simulink model "visual_line_follower_sac_lyapunov_gazebo"  (R2026a)
settings: Solver=FixedStepDiscrete  StopTime=inf  FixedStep=Ts_Control  EnableMultiTasking=on
InitFcn:
  | run(fullfile(fileparts(get_param(bdroot,"FileName")),"runtime","configure_visual_line_follower_gazebo_debug.m"));
model workspace (MAT data in the model file):
  BaseLinearSpeed = 20
  BaseSpeedScale = 0.03
  Kd_Line = 0.35
  Ki_Line = 0
  Kp_Line = 5
  LocalPath_CurvatureGain = 0.04
  LocalPath_HeadingGain = 0.35
  LocalPath_LateralGain = 0.6
  LocalPath_LookaheadDistance = 0.72
  LocalPath_NumPoints = 30
  LocalPath_ROIFraction = 0.1
  MJ_StepTime = 0.002
  MJ_TargetLateralPosition = 0
  MaxAngularSpeed = 1.5
  MaxWheelSpeed = 25
  N_Line = 20
  OriginBot_ErrorScale = 500
  OriginBot_MaxSaturation = 0.3
  OriginBot_MinBrightness = 70
  OriginBot_MinPixels = 30
  OriginBot_ROIHeight = 45
  OriginBot_ROIStartFraction = 0.72
  SAC_Done_Steps = 100
  SAC_Eps = 0.001
  SAC_K_inv = 0.1
  SAC_Lambda = 0.5
  SAC_MaxDeltaOmega = 1
  SAC_P_Lost = 10
  SAC_Q = 1
  SAC_Q_e = 1
  SAC_Q_h = 1
  SAC_Q_l = 1
  SAC_R = 0.1
  SL_ROS_VariableLengthArrays_MaxSizes.CommonInfo.ArrayTruncateAction = 'EmitWarning'
  SL_ROS_VariableLengthArrays_MaxSizes.MsgTypeMap = containers.Map
  SL_ROS_VariableLengthArrays_MaxSizes.MsgTypeMap.serialization.keys = {'sensor_msgs/Image'}
  SL_ROS_VariableLengthArrays_MaxSizes.MsgTypeMap.serialization.values{1}(1).PropertyName = 'data'
  SL_ROS_VariableLengthArrays_MaxSizes.MsgTypeMap.serialization.values{1}(1).DataType = 'uint8'
  SL_ROS_VariableLengthArrays_MaxSizes.MsgTypeMap.serialization.values{1}(1).MaxLength = 6220800
  SL_ROS_VariableLengthArrays_MaxSizes.MsgTypeMap.serialization.values{1}(2).PropertyName = 'encoding'
  SL_ROS_VariableLengthArrays_MaxSizes.MsgTypeMap.serialization.values{1}(2).DataType = 'uint8'
  SL_ROS_VariableLengthArrays_MaxSizes.MsgTypeMap.serialization.values{1}(2).MaxLength = 128
  SL_ROS_VariableLengthArrays_MaxSizes.MsgTypeMap.serialization.uniformity = 0
  SL_ROS_VariableLengthArrays_MaxSizes.MsgTypeMap.serialization.keyType = 'char'
  SL_ROS_VariableLengthArrays_MaxSizes.MsgTypeMap.serialization.valueType = 'any'
  SteeringSign = 1
  TB3_WheelRadius = 0.033
  TB3_WheelSeparation = 0.288
  Ts_Control = 0.05
  Ts_Stop = 10
  Ts_Vision = 0.05
  TurtleBot3MuJoCoMap = "complex"
  TurtleBot3MuJoCoScene = ""
  k_heading = 0.55
undefined symbols (not defined in the file): angular, linear, originbot_line_follower_debug_frame_gazebo, originbot_local_path_generator_gazebo
libraries: ros2lib x4, slpidlib x1, rllib x1
settings Model: ExtModeTrigDuration=10000  Creator=HP  LastModifiedBy=kevin
settings SolverCC: PositivePriorityOrder=on
settings ConfigComp: CovMetricSettings=dswe

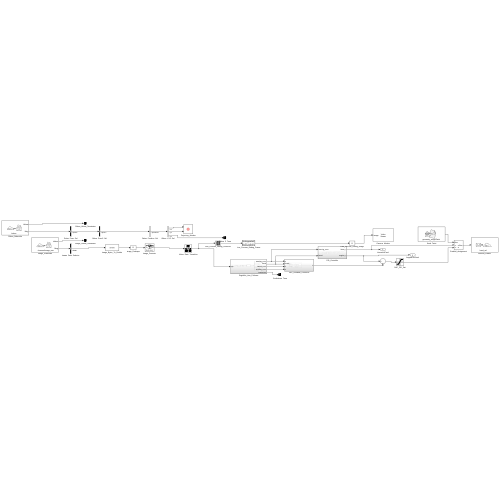
[thumbnail: Simulink's stored preview of the top-level diagram]
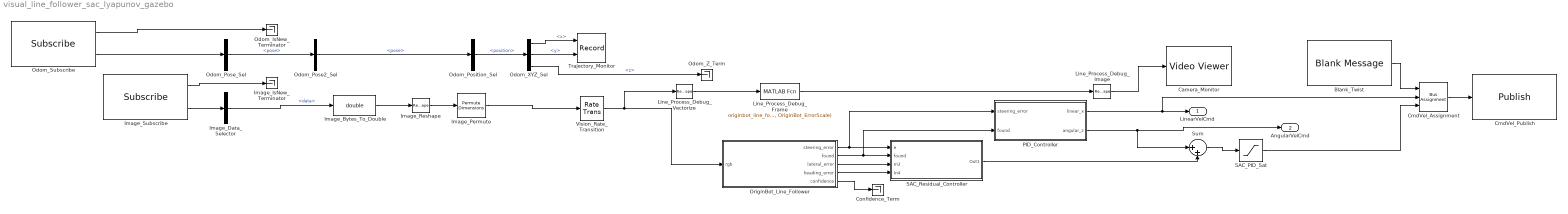
== system visual_line_follower_sac_lyapunov_gazebo ==
  Blank_Twist : ros2lib/Blank Message  messageClass=Message  entityType=geometry_msgs/Twist  messageType=geometry_msgs/Twist  SampleTime=inf
  Camera_Monitor : VideoViewer  FigPos=[2041 741 418 304]
  CmdVel_Assignment : BusAssignment  AssignedSignals=linear.x,angular.z
  CmdVel_Publish : ros2lib/Publish  topicSource=Select from ROS network  topic=/cmd_vel  messageType=geometry_msgs/Twist  QOSHistory=Keep last  QOSDepth=10  QOSReliability=Reliable  QOSDurability=Volatile  QOSDeadline=Inf  QOSLifespan=Inf  QOSLiveliness=Automatic  QOSLeaseDuration=Inf  QOSAvoidROSNamespaceConventions=off
  Confidence_Term : Terminator
  Image_Bytes_To_Double : DataTypeConversion  OutDataTypeStr=double
  Image_Data_Selector : BusSelector  OutputSignals=data
  Image_IsNew_Terminator : Terminator
  Image_Permute : PermuteDimensions  Order=[3 2 1]
  Image_Reshape : Reshape  OutputDimensionality=Customize  OutputDimensions=[3,1920,1080]
  Image_Subscribe : ros2lib/Subscribe  topicSource=Select from ROS network  topic=/camera/image_raw  messageType=sensor_msgs/Image  sampleTime=Ts_Vision  QOSHistory=Keep last  QOSDepth=10  QOSReliability=Reliable  QOSDurability=Volatile  QOSDeadline=Inf  QOSLifespan=Inf  QOSLiveliness=Automatic  QOSLeaseDuration=Inf  QOSAvoidROSNamespaceConventions=off
  Line_Process_Debug_Frame : MATLABFcn  MATLABFcn=originbot_line_follower_debug_frame_gazebo(u, LocalPath_ROIFraction, LocalPath_NumPoints, OriginBot_MinBrightness, OriginBot_MaxSaturation, OriginBot_MinPixels, OriginBot_ErrorScale)
  Line_Process_Debug_Image : Reshape  OutputDimensionality=Customize  OutputDimensions=[1080,1920,3]
  Line_Process_Debug_Vectorize : Reshape  OutputDimensionality=Column vector (2-D)
  Odom_IsNew_Terminator : Terminator
  Odom_Pose2_Sel : BusSelector  OutputSignals=pose
  Odom_Pose_Sel : BusSelector  OutputSignals=pose
  Odom_Position_Sel : BusSelector  OutputSignals=position
  Odom_Subscribe : ros2lib/Subscribe  topicSource=Select from ROS network  topic=/odom  messageType=nav_msgs/Odometry  sampleTime=Ts_Control  QOSHistory=Keep last  QOSDepth=10  QOSReliability=Reliable  QOSDurability=Volatile  QOSDeadline=Inf  QOSLifespan=Inf  QOSLiveliness=Automatic  QOSLeaseDuration=Inf  QOSAvoidROSNamespaceConventions=off
  Odom_XYZ_Sel : BusSelector  OutputSignals=x,y,z
  Odom_Z_Term : Terminator
  OriginBot_Line_Follower : Subsystem
  PID_Controller : Subsystem
  SAC_PID_Sat : Saturate  UpperLimit=2*MaxWheelSpeed*TB3_WheelRadius/TB3_WheelSeparation  LowerLimit=-2*MaxWheelSpeed*TB3_WheelRadius/TB3_WheelSeparation
  SAC_Residual_Controller : Subsystem
  Sum : Sum  Inputs=|++
  Trajectory_Monitor : Record  NumPorts=2.0  FileSettingsInternal="{\"entries\":[{\"content\":{\"excelSettings\":{\"content\":{},\"type\":\"Streamout.ExcelSettings\"},\"parquetSettings\":{\"content\":{},\"type\":\"Streamout.ParquetSettings\"}},\"type\":\"Streamout.FileSettingStorage\",\"uuid\":\"\"}],\"packageUris\":[\"http:\\/\\/schema.mathworks.com\\/mf0\\/streamout_blocks\\/R2020a\"],\"version\":\"1.0\"}"  FrameSettings=[0, 0]  SignalsInternal="{\"entries\":[{\"content\":{},\"type\":\"RecordBlkView.InputSignals\",\"uuid\":\"\"}],\"packageUris\":[\"http:\\/\\/schema.mathworks.com\\/mf0\\/streamout_blocks\\/R2020a\"],\"version\":\"1.0\"}"  VisualizationBindings="{\"sparklinesplugin\":{\"info\":[{\"bindingParametersList\":[],\"subplotID\":1}]}}"
  Vision_Rate_Transition : RateTransition
  LinearVelCmd : Outport
  AngularVelCmd : Outport  Port=2
  wires:
  SAC_PID_Sat/1 -> CmdVel_Assignment/3
  Line_Process_Debug_Image/1 -> Camera_Monitor/1
  Line_Process_Debug_Frame/1 -> Line_Process_Debug_Image/1
  Line_Process_Debug_Vectorize/1 -> Line_Process_Debug_Frame/1
  Image_Permute/1 -> Vision_Rate_Transition/1
  Image_Reshape/1 -> Image_Permute/1
  Image_Bytes_To_Double/1 -> Image_Reshape/1
  Image_Data_Selector/1 -> Image_Bytes_To_Double/1  "<data>"
  Image_Subscribe/2 -> Image_Data_Selector/1
  Image_Subscribe/1 -> Image_IsNew_Terminator/1
  Sum/1 -> SAC_PID_Sat/1
  SAC_Residual_Controller/1(Out1) -> Sum/2
  PID_Controller/2(angular_z) -> Sum/1, AngularVelCmd/1
  PID_Controller/1(linear_x) -> LinearVelCmd/1, CmdVel_Assignment/2
  Blank_Twist/1 -> CmdVel_Assignment/1
  CmdVel_Assignment/1 -> CmdVel_Publish/1
  Odom_Subscribe/1 -> Odom_IsNew_Terminator/1
  Odom_Subscribe/2 -> Odom_Pose_Sel/1
  Odom_Pose_Sel/1 -> Odom_Pose2_Sel/1  "<pose>"
  Odom_Pose2_Sel/1 -> Odom_Position_Sel/1  "<pose>"
  Odom_Position_Sel/1 -> Odom_XYZ_Sel/1  "<position>"
  Odom_XYZ_Sel/3 -> Odom_Z_Term/1  "<z>"
  Odom_XYZ_Sel/1 -> Trajectory_Monitor/1  "<x>"
  Odom_XYZ_Sel/2 -> Trajectory_Monitor/2  "<y>"
  Vision_Rate_Transition/1 -> OriginBot_Line_Follower/1(rgb), Line_Process_Debug_Vectorize/1
  OriginBot_Line_Follower/1(steering_error) -> SAC_Residual_Controller/1(e), PID_Controller/1(steering_error)
  OriginBot_Line_Follower/2(found) -> SAC_Residual_Controller/2(found), PID_Controller/2(found)
  OriginBot_Line_Follower/3(lateral_error) -> SAC_Residual_Controller/3(In3)
  OriginBot_Line_Follower/4(heading_error) -> SAC_Residual_Controller/4(In4)
  OriginBot_Line_Follower/5(confidence) -> Confidence_Term/1

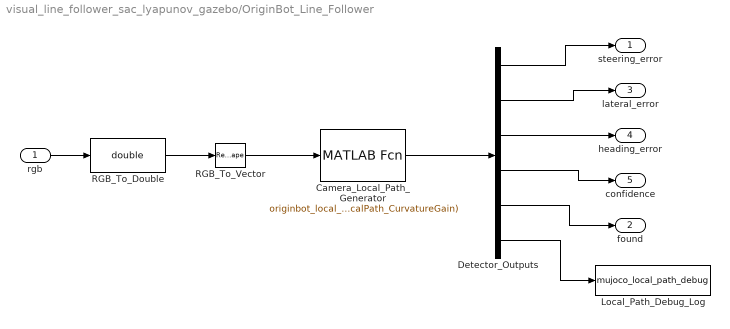
== system visual_line_follower_sac_lyapunov_gazebo/OriginBot_Line_Follower ==
  rgb : Inport
  Camera_Local_Path_Generator : MATLABFcn  MATLABFcn=originbot_local_path_generator_gazebo(u, LocalPath_ROIFraction, LocalPath_NumPoints, OriginBot_MinBrightness, OriginBot_MaxSaturation, OriginBot_MinPixels, OriginBot_ErrorScale, LocalPath_LookaheadDistance, LocalPath_LateralGain, LocalPath_HeadingGain, LocalPath_CurvatureGain)  OutputDimensions=72  OutputSignalType=real  SampleTime=Ts_Vision
  Detector_Outputs : Demux  Outputs=[1 1 1 1 1 67]
  Local_Path_Debug_Log : ToWorkspace  VariableName=mujoco_local_path_debug  SaveFormat=Timeseries  SampleTime=-1
  RGB_To_Double : DataTypeConversion  OutDataTypeStr=double
  RGB_To_Vector : Reshape  OutputDimensionality=Column vector (2-D)
  steering_error : Outport
  found : Outport  Port=2
  lateral_error : Outport  Port=3
  heading_error : Outport  Port=4
  confidence : Outport  Port=5
  wires:
  Detector_Outputs/6 -> Local_Path_Debug_Log/1
  Detector_Outputs/5 -> found/1
  Detector_Outputs/3 -> heading_error/1
  Detector_Outputs/1 -> steering_error/1
  Camera_Local_Path_Generator/1 -> Detector_Outputs/1
  Detector_Outputs/4 -> confidence/1
  RGB_To_Vector/1 -> Camera_Local_Path_Generator/1
  RGB_To_Double/1 -> RGB_To_Vector/1
  rgb/1 -> RGB_To_Double/1
  Detector_Outputs/2 -> lateral_error/1

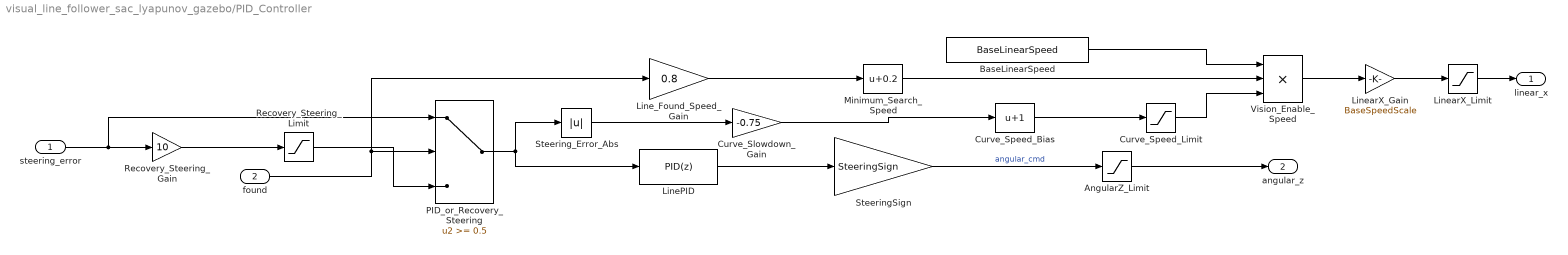
== system visual_line_follower_sac_lyapunov_gazebo/PID_Controller ==
  steering_error : Inport
  found : Inport  Port=2
  AngularZ_Limit : Saturate  UpperLimit=2*MaxWheelSpeed*TB3_WheelRadius/TB3_WheelSeparation  LowerLimit=-2*MaxWheelSpeed*TB3_WheelRadius/TB3_WheelSeparation
  BaseLinearSpeed : Constant  Value=BaseLinearSpeed
  Curve_Slowdown_Gain : Gain  Gain=-0.75
  Curve_Speed_Bias : Bias  Bias=1
  Curve_Speed_Limit : Saturate  UpperLimit=1  LowerLimit=0.25
  LinePID : slpidlib/PID Controller  Controller=PID  Form=Parallel  TimeDomain=Discrete-time  UseExternalTs=off  SampleTime=Ts_Control  IntegratorMethod=Backward Euler  FilterMethod=Trapezoidal  ControllerParametersSource=internal  P=Kp_Line  I=Ki_Line  UseKiTs=off  D=Kd_Line  UseExternalDerivativeSource=off  N=N_Line  UseFilter=on  TunerSelectOption=Transfer Function Based (PID Tuner App)  InitialConditionSource=internal  InitialConditionForIntegrator=0  InitialConditionForFilter=0  DifferentiatorICPrevScaledInput=0  ExternalReset=none  TrackingMode=off  Kt=1  LimitOutput=on  SatLimitsSource=internal  UpperSaturationLimit=MaxAngularSpeed  LowerSaturationLimit=-MaxAngularSpeed  LinearizeAsGain=off  AntiWindupMode=back-calculation  Kb=1  LimitIntegrator=off  UpperIntegratorSaturationLimit=inf  LowerIntegratorSaturationLimit=-inf  POutMin=[]  POutMax=[]  IOutMin=[]  IOutMax=[]  DOutMin=[]  DOutMax=[]  NOutMin=[]  NOutMax=[]  SumOutMin=[]  SumOutMax=[]  SaturationOutMin=[]  SaturationOutMax=[]  PParamMin=[]  PParamMax=[]  IParamMin=[]  IParamMax=[]  DParamMin=[]  DParamMax=[]  NParamMin=[]  NParamMax=[]  KbParamMin=[]  KbParamMax=[]  KtParamMin=[]  KtParamMax=[]  KbOutMin=[]  KbOutMax=[]  KtOutMin=[]  KtOutMax=[]  IntegratorOutMin=[]  IntegratorOutMax=[]  FilterOutMin=[]  FilterOutMax=[]  SumI1OutMin=[]  SumI1OutMax=[]  SumI2OutMin=[]  SumI2OutMax=[]  SumI3OutMin=[]  SumI3OutMax=[]  SumI4OutMin=[]  SumI4OutMax=[]  SumDOutMin=[]  SumDOutMax=[]  DifferentiatorOutMin=[]  DifferentiatorOutMax=[]  FilterDiffOutCoefMin=[]  FilterDiffOutCoefMax=[]  ReciprocalOutMin=[]  ReciprocalOutMax=[]  SumDenOutMin=[]  SumDenOutMax=[]  SumNumOutMin=[]  SumNumOutMax=[]  DivideOutMin=[]  DivideOutMax=[]  UdiffTsProdOutMin=[]  UdiffTsProdOutMax=[]  NTsProdOutMin=[]  NTsProdOutMax=[]  UintegralTsProdOutMin=[]  UintegralTsProdOutMax=[]  UngainTsProdOutMin=[]  UngainTsProdOutMax=[]  ClampingZeroOutDataTypeStr=Inherit: Inherit via back propagation  ClampingZeroOutMin=[]  ClampingZeroOutMax=[]  FilterDenConstantOutDataTypeStr=Inherit: Inherit via back propagation  FilterDenConstantOutMin=[]  FilterDenConstantOutMax=[]  PCopyOutDataTypeStr=Inherit: Inherit via back propagation  PCopyOutMin=[]  PCopyOutMax=[]  NCopyOutDataTypeStr=Inherit: Inherit via back propagation  NCopyOutMin=[]  NCopyOutMax=[]  IntegratorContinuousStateAttributes=''  IntegratorStateMustResolveToSignalObject=off  IntegratorRTWStateStorageClass=Auto  FilterContinuousStateAttributes=''  FilterStateMustResolveToSignalObject=off  FilterRTWStateStorageClass=Auto  ParallelPVariant=InternalParameters  IdealPVariant=Disabled  IVariant=InternalParameters  DVariant=InternalParameters  IntegratorVariant=Discrete  SatVariant=Enabled  AWVariant=BackCalculation  PCopyVariant=Disabled  TRVariant=Disabled  FdbkBlocksVariant=Feedback  IdealPFdbkVariant=Passthrough  SatFdbkVariant=Enabled  DerivativeFilterVariant=TrapezoidalFilter  NVariant=InternalParameters  NCopyVariant=InternalParameters  FilterICVariant=InternalICsFilter  IntegratorICVariant=InternalICs  ExternalResetVariant=Disabled  TRSumVariant=Passthrough  SumFdbkVariant=Enabled  SumVariant=Sum_PID  TsampFilterVariant=InternalTs  TsampNgainVariant=Passthrough  TsampIntegralVariant=Disabled_SignalSpec  ExternalSaturationOutDataTypeStr=Inherit: Same as second input  DerivativeSourceVariant=ErrorSignal  PreIntVariant=InternalPreInt
      settings: LibrarySourceBlock=hdlsllib/Discrete/Discrete PID Controller
  Line_Found_Speed_Gain : Gain  Gain=0.8
  LinearX_Gain : Gain  Gain=BaseSpeedScale
  LinearX_Limit : Saturate  UpperLimit=MaxWheelSpeed*TB3_WheelRadius  LowerLimit=-MaxWheelSpeed*TB3_WheelRadius
  Minimum_Search_Speed : Bias  Bias=0.2
  PID_or_Recovery_Steering : Switch  Threshold=0.5
  Recovery_Steering_Gain : Gain  Gain=10
  Recovery_Steering_Limit : Saturate  UpperLimit=0.45  LowerLimit=-0.45
  SteeringSign : Gain  Gain=SteeringSign
  Steering_Error_Abs : Abs
  Vision_Enable_Speed : Product  Inputs=***
  linear_x : Outport
  angular_z : Outport  Port=2
  wires:
  AngularZ_Limit/1 -> angular_z/1
  SteeringSign/1 -> AngularZ_Limit/1  "angular_cmd"
  LinearX_Limit/1 -> linear_x/1
  LinearX_Gain/1 -> LinearX_Limit/1
  Vision_Enable_Speed/1 -> LinearX_Gain/1
  Curve_Speed_Limit/1 -> Vision_Enable_Speed/3
  BaseLinearSpeed/1 -> Vision_Enable_Speed/1
  LinePID/1 -> SteeringSign/1
  Curve_Speed_Bias/1 -> Curve_Speed_Limit/1
  Curve_Slowdown_Gain/1 -> Curve_Speed_Bias/1
  Steering_Error_Abs/1 -> Curve_Slowdown_Gain/1
  Line_Found_Speed_Gain/1 -> Minimum_Search_Speed/1
  Recovery_Steering_Limit/1 -> PID_or_Recovery_Steering/3
  Recovery_Steering_Gain/1 -> Recovery_Steering_Limit/1
  PID_or_Recovery_Steering/1 -> LinePID/1, Steering_Error_Abs/1
  found/1 -> PID_or_Recovery_Steering/2, Line_Found_Speed_Gain/1
  Minimum_Search_Speed/1 -> Vision_Enable_Speed/2
  steering_error/1 -> PID_or_Recovery_Steering/1, Recovery_Steering_Gain/1

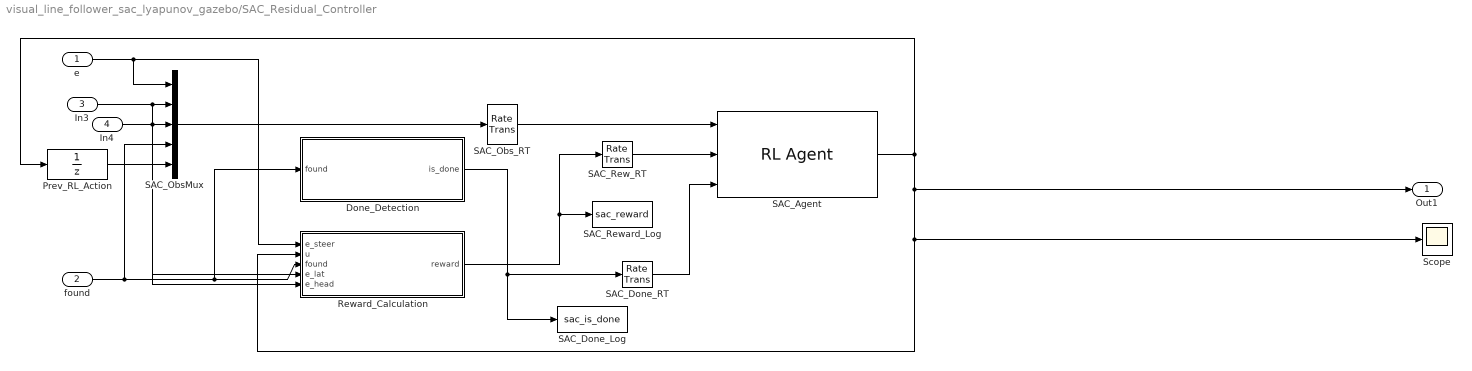
== system visual_line_follower_sac_lyapunov_gazebo/SAC_Residual_Controller ==
  e : Inport
  found : Inport  Port=2
  In3 : Inport  Port=3
  In4 : Inport  Port=4
  Done_Detection : Subsystem
  Prev_RL_Action : UnitDelay  SampleTime=Ts_Control
  Reward_Calculation : Subsystem
  SAC_Agent : rllib/RL Agent  Agent=trainedAgent  ExternalActionAsInput=off  ProvideLastAction=off  ProvideCumRwd=off  TreatAsDirectFeedthrough=on  UseStrictObservationDataTypes=off
  SAC_Done_Log : ToWorkspace  VariableName=sac_is_done  SaveFormat=Timeseries  SampleTime=-1
  SAC_Done_RT : RateTransition  Integrity=off  Deterministic=off
  SAC_ObsMux : Mux  Inputs=5
  SAC_Obs_RT : RateTransition  Integrity=off  Deterministic=off
  SAC_Rew_RT : RateTransition  Integrity=off  Deterministic=off
  SAC_Reward_Log : ToWorkspace  VariableName=sac_reward  SaveFormat=Timeseries  SampleTime=-1
  Scope : Scope
      settings: ActiveDisplayYMinimum=-1  ActiveDisplayYMaximum=1
  Out1 : Outport
  wires:
  e/1 -> Reward_Calculation/1(e_steer), SAC_ObsMux/1
  found/1 -> Done_Detection/1(found), Reward_Calculation/3(found), SAC_ObsMux/4
  SAC_Rew_RT/1 -> SAC_Agent/2
  SAC_Done_RT/1 -> SAC_Agent/3
  SAC_Obs_RT/1 -> SAC_Agent/1
  SAC_Agent/1 -> Scope/1, Reward_Calculation/2(u), Out1/1, Prev_RL_Action/1
  In3/1 -> SAC_ObsMux/2, Reward_Calculation/4(e_lat)
  In4/1 -> SAC_ObsMux/3, Reward_Calculation/5(e_head)
  Prev_RL_Action/1 -> SAC_ObsMux/5
  SAC_ObsMux/1 -> SAC_Obs_RT/1
  Reward_Calculation/1(reward) -> SAC_Rew_RT/1, SAC_Reward_Log/1
  Done_Detection/1(is_done) -> SAC_Done_Log/1, SAC_Done_RT/1

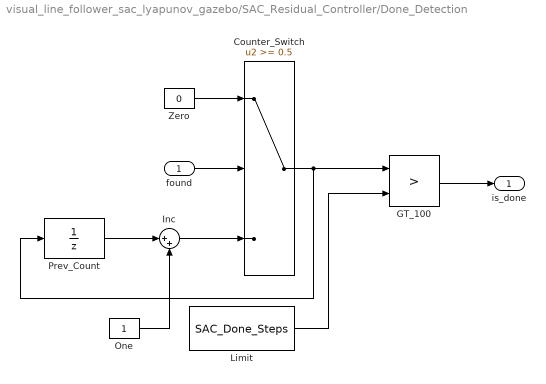
== system visual_line_follower_sac_lyapunov_gazebo/SAC_Residual_Controller/Done_Detection ==
  found : Inport
  Counter_Switch : Switch  Threshold=0.5  SaturateOnIntegerOverflow=off  InputSameDT=off
  GT_100 : RelationalOperator  Operator=>  OutDataTypeStr=boolean  RndMeth=Simplest  InputSameDT=off
  Inc : Sum  Inputs=|++
  Limit : Constant  Value=SAC_Done_Steps
  One : Constant
  Prev_Count : UnitDelay  SampleTime=Ts_Control
  Zero : Constant  Value=0
  is_done : Outport
  wires:
  Prev_Count/1 -> Inc/1
  One/1 -> Inc/2
  found/1 -> Counter_Switch/2
  Zero/1 -> Counter_Switch/1
  GT_100/1 -> is_done/1
  Inc/1 -> Counter_Switch/3
  Limit/1 -> GT_100/2
  Counter_Switch/1 -> Prev_Count/1, GT_100/1

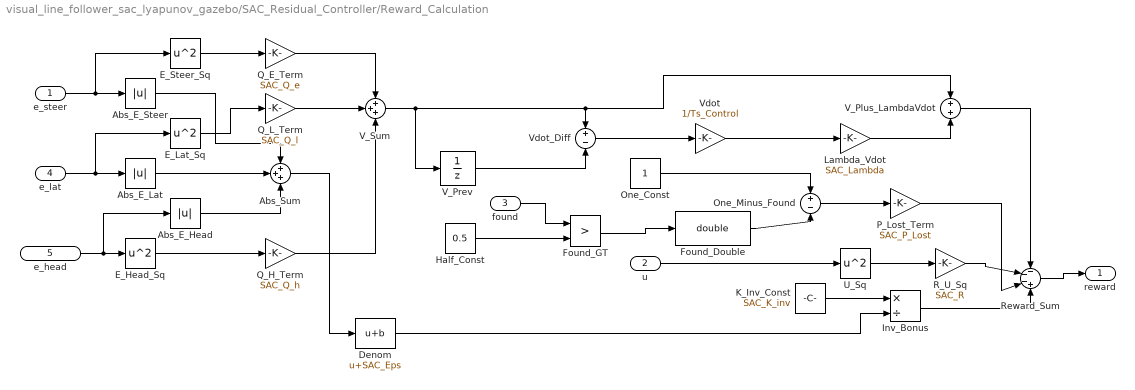
== system visual_line_follower_sac_lyapunov_gazebo/SAC_Residual_Controller/Reward_Calculation ==
  e_steer : Inport
  u : Inport  Port=2
  found : Inport  Port=3
  e_lat : Inport  Port=4
  e_head : Inport  Port=5
  Abs_E_Head : Abs
  Abs_E_Lat : Abs
  Abs_E_Steer : Abs
  Abs_Sum : Sum  Inputs=+++
  Denom : Bias  Bias=SAC_Eps
  E_Head_Sq : Math  Operator=square
  E_Lat_Sq : Math  Operator=square
  E_Steer_Sq : Math  Operator=square
  Found_Double : DataTypeConversion  OutDataTypeStr=double
  Found_GT : RelationalOperator  Operator=>
  Half_Const : Constant  Value=0.5
  Inv_Bonus : Product  Inputs=*/
  K_Inv_Const : Constant  Value=SAC_K_inv
  Lambda_Vdot : Gain  Gain=SAC_Lambda
  One_Const : Constant
  One_Minus_Found : Sum  Inputs=+-
  P_Lost_Term : Gain  Gain=SAC_P_Lost
  Q_E_Term : Gain  Gain=SAC_Q_e
  Q_H_Term : Gain  Gain=SAC_Q_h
  Q_L_Term : Gain  Gain=SAC_Q_l
  R_U_Sq : Gain  Gain=SAC_R
  Reward_Sum : Sum  Inputs=---+
  U_Sq : Math  Operator=square
  V_Plus_LambdaVdot : Sum
  V_Prev : UnitDelay  SampleTime=Ts_Control
  V_Sum : Sum  Inputs=+++
  Vdot : Gain  Gain=1/Ts_Control
  Vdot_Diff : Sum  Inputs=+-
  reward : Outport
  wires:
  One_Minus_Found/1 -> P_Lost_Term/1
  Found_Double/1 -> One_Minus_Found/2
  One_Const/1 -> One_Minus_Found/1
  Found_GT/1 -> Found_Double/1
  Half_Const/1 -> Found_GT/2
  found/1 -> Found_GT/1
  U_Sq/1 -> R_U_Sq/1
  u/1 -> U_Sq/1
  e_steer/1 -> Abs_E_Steer/1, E_Steer_Sq/1
  e_lat/1 -> E_Lat_Sq/1, Abs_E_Lat/1
  e_head/1 -> Abs_E_Head/1, E_Head_Sq/1
  E_Steer_Sq/1 -> Q_E_Term/1
  E_Lat_Sq/1 -> Q_L_Term/1
  E_Head_Sq/1 -> Q_H_Term/1
  Q_E_Term/1 -> V_Sum/1
  Q_L_Term/1 -> V_Sum/2
  Q_H_Term/1 -> V_Sum/3
  V_Sum/1 -> V_Plus_LambdaVdot/1, Vdot_Diff/1, V_Prev/1
  V_Prev/1 -> Vdot_Diff/2
  Vdot_Diff/1 -> Vdot/1
  Vdot/1 -> Lambda_Vdot/1
  Lambda_Vdot/1 -> V_Plus_LambdaVdot/2
  Abs_E_Steer/1 -> Abs_Sum/1
  Abs_E_Lat/1 -> Abs_Sum/2
  Abs_E_Head/1 -> Abs_Sum/3
  Abs_Sum/1 -> Denom/1
  K_Inv_Const/1 -> Inv_Bonus/1
  Denom/1 -> Inv_Bonus/2
  V_Plus_LambdaVdot/1 -> Reward_Sum/1
  R_U_Sq/1 -> Reward_Sum/2
  P_Lost_Term/1 -> Reward_Sum/3
  Inv_Bonus/1 -> Reward_Sum/4
  Reward_Sum/1 -> reward/1
